simulink model "chap7_9sim"  (Simulink 8.1)
settings: Solver=ode45  StartTime=0.0  StopTime=20  FixedStep=0.001  RelTol=1e-3  AbsTol=1e-3
settings Model: Creator=ThinkPad  LastModifiedBy=liujk  ExtModeTrigMode=oneshot  ExtModeArmWhenConnect=off
settings DataIOCC: LimitDataPoints=off  SignalLoggingName=sigsOut
settings OptimizationCC: BooleanDataType=off  InitFltsAndDblsToZero=on
settings DebuggingCC: SaveWithParameterizedLinksMsg=none  SignalResolutionControl=TryResolveAllWithWarning  SolverPrmCheckMsg=none  MultiTaskDSMMsg=warning  MultiTaskCondExecSysMsg=none  StrictBusMsg=None
settings HardwareCC: TargetUnknown=on
settings RTWCC: IncludeERTFirstTime=on
settings GRTTargetCC: TargetFcnLib=ansi_tfl_tmw.mat

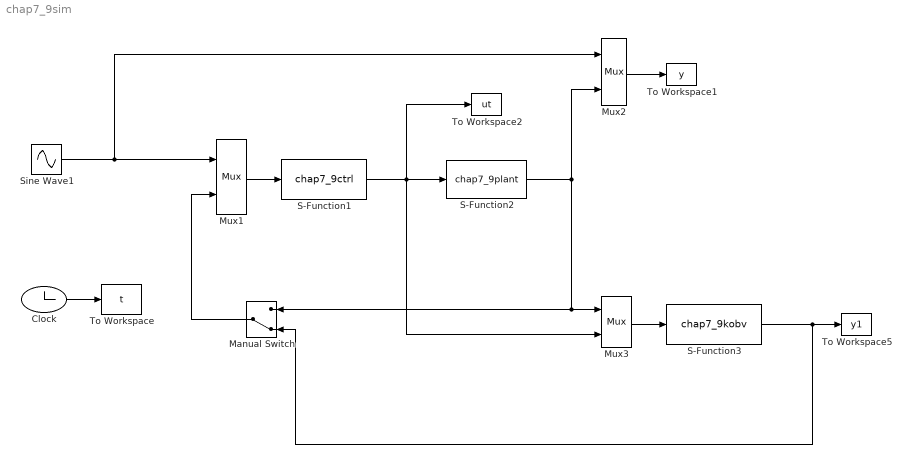
== system chap7_9sim ==
  Clock : Clock
  Manual Switch : ManualSwitch  CurrentSetting=0
  Mux1 : Mux  Inputs=2
  Mux2 : Mux  Inputs=2
  Mux3 : Mux  Inputs=2
  S-Function1 : S-Function  FunctionName=chap7_9ctrl  EnableBusSupport=off
  S-Function2 : S-Function  FunctionName=chap7_9plant  EnableBusSupport=off
  S-Function3 : S-Function  FunctionName=chap7_9kobv  EnableBusSupport=off
  Sine Wave1 : Sin  SampleTime=0
  To Workspace : ToWorkspace  VariableName=t  SampleTime=-1
  To Workspace1 : ToWorkspace  VariableName=y  SampleTime=-1
  To Workspace2 : ToWorkspace  VariableName=ut  SampleTime=-1
  To Workspace5 : ToWorkspace  VariableName=y1  SampleTime=-1
  wires:
  Clock/1 -> To Workspace/1
  Mux2/1 -> To Workspace1/1
  S-Function1/1 -> Mux3/2, S-Function2/1, To Workspace2/1
  Mux1/1 -> S-Function1/1
  Sine Wave1/1 -> Mux2/1, Mux1/1
  Manual Switch/1 -> Mux1/2
  Mux3/1 -> S-Function3/1
  S-Function3/1 -> Manual Switch/2, To Workspace5/1
  S-Function2/1 -> Manual Switch/1, Mux3/1, Mux2/2
